simulink model "pwm_fpga"  (R2020b)
settings: Solver=FixedStepDiscrete  StartTime=0.0  StopTime=5  FixedStep=1e-3  RelTol=1e-3
PostLoadFcn:
  | try
  | cell = struct2cell(dir(fullfile(speedgoatroot_hdlb, 'hdlsrc', 'pwm', '*.vhd')));
  | addSourceFiles = strjoin(fullfile(cell(2,:),cell(1,:)), ';');
  | hdlset_param('pwm_example_hdlc/DUT PWM and CAP', 'IPCoreAdditionalFiles', addSourceFiles);
  | end
libraries: pwm_fpgalib x1, pwm_cpulib x1
settings Model: ModifiedByFormat=Speedgoat GmbH  Creator=Speedgoat GmbH  LastModifiedBy=Speedgoat GmbH
settings DataIOCC: LimitDataPoints=on  SaveFormat=Array  ReturnWorkspaceOutputs=off
settings OptimizationCC: BlockReduction=off  ConditionallyExecuteInputs=off  DefaultParameterBehavior=Inlined  LifeSpan=inf
settings DebuggingCC: AlgebraicLoopMsg=error  UnderspecifiedInitializationDetection=Classic  MergeDetectMultiDrivingBlocksExec=none  SolverPrmCheckMsg=warning  SingleTaskRateTransMsg=error  PregeneratedLibrarySubsystemCodeDiagnostic=none  SFUnexpectedBacktrackingDiag=warning  SFNoUnconditionalDefaultTransitionDiag=warning  SFExecutionAtInitializationDiag=none  ArithmeticOperatorsInVariantConditions=warning
settings HardwareCC: ProdBitPerPointer=32  ProdBitPerSizeT=32  ProdBitPerPtrDiffT=32  ProdLargestAtomicFloat=None  ProdIntDivRoundTo=Undefined  ProdEndianess=Unspecified  ProdWordSize=32  ProdHWDeviceType=ASIC/FPGA->ASIC/FPGA  ProdEqTarget=off
settings ModelReferenceCC: PropagateSignalLabelsOutOfModel=off
settings SFSimCC: SimUseLocalCustomCode=off  CustomCodeUndefinedFunction=UseInterfaceOnly
settings RTWCC: RTWUseLocalCustomCode=off
settings CodeAppCC: StateflowObjectComments=on
settings GRTTargetCC: TargetLangStandard=C89/C90 (ANSI)
settings ConfigComp: CovMetricSettings=dw  CovSaveCumulativeToWorkspaceVar=on  CovSaveSingleToWorkspaceVar=on  CovExternalEMLEnable=off

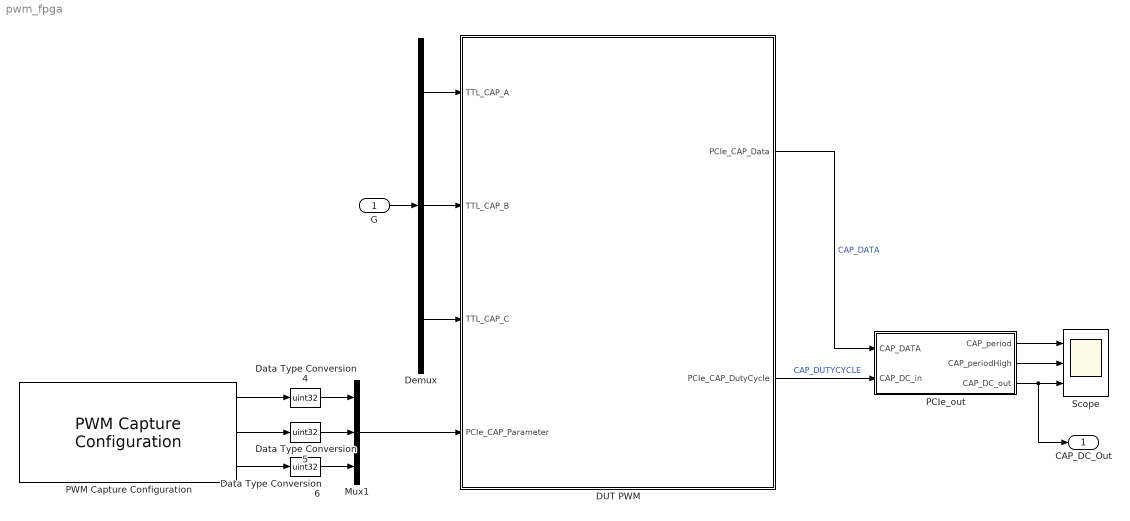
== system pwm_fpga ==
  G : Inport
  DUT PWM : Subsystem
  Data Type Conversion4 : DataTypeConversion  OutDataTypeStr=uint32
  Data Type Conversion5 : DataTypeConversion  OutDataTypeStr=uint32
  Data Type Conversion6 : DataTypeConversion  OutDataTypeStr=uint32
  Demux : Demux  Outputs=3
  Mux1 : Mux  Inputs=3
  PCIe_out : Subsystem
  PWM Capture Configuration : pwm_cpulib/PWM Capture Configuration  FPGA_freq=100e6  n_channels=1  captureMode=High transitions triggered  captureTimeout=0  PWM_pattern_en=off
      settings: SourceProductName=Simulink Real-Time: Speedgoat HDL Blockset
  Scope : Scope  NumInputPorts=3
  CAP_DC_Out : Outport  VectorParamsAs1DForOutWhenUnconnected=off
  wires:
  DUT PWM/2(PCIe_CAP_DutyCycle) -> PCIe_out/2(CAP_DC_in)  "CAP_DUTYCYCLE"
  DUT PWM/1(PCIe_CAP_Data) -> PCIe_out/1(CAP_DATA)  "CAP_DATA"
  PCIe_out/3(CAP_DC_out) -> Scope/3, CAP_DC_Out/1
  PCIe_out/2(CAP_periodHigh) -> Scope/2
  PCIe_out/1(CAP_period) -> Scope/1
  PWM Capture Configuration/1 -> Data Type Conversion4/1
  PWM Capture Configuration/3 -> Data Type Conversion6/1
  PWM Capture Configuration/2 -> Data Type Conversion5/1
  Data Type Conversion4/1 -> Mux1/1
  Data Type Conversion5/1 -> Mux1/2
  Data Type Conversion6/1 -> Mux1/3
  Mux1/1 -> DUT PWM/4(PCIe_CAP_Parameter)
  Demux/1 -> DUT PWM/1(TTL_CAP_A)
  Demux/3 -> DUT PWM/3(TTL_CAP_C)
  Demux/2 -> DUT PWM/2(TTL_CAP_B)
  G/1 -> Demux/1

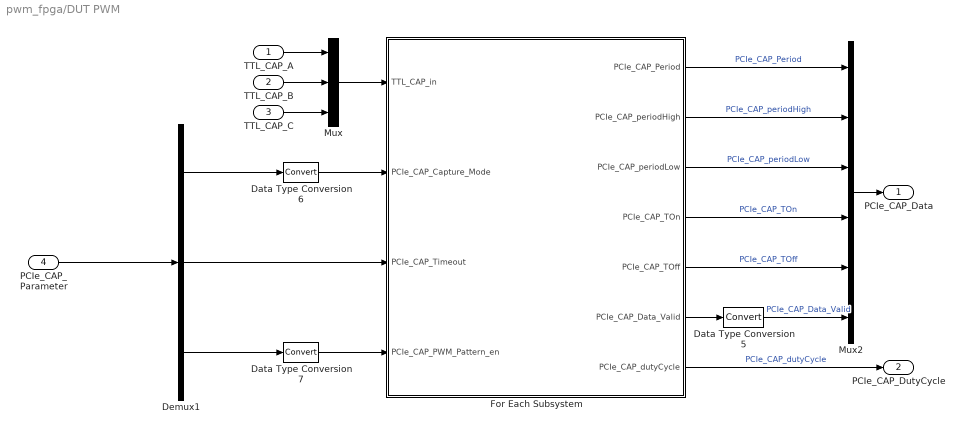
== system pwm_fpga/DUT PWM ==
  TTL_CAP_A : Inport
  TTL_CAP_B : Inport  Port=2
  TTL_CAP_C : Inport  Port=3
  PCIe_CAP_Parameter : Inport  Port=4
  Data Type Conversion5 : DataTypeConversion
  Data Type Conversion6 : DataTypeConversion
  Data Type Conversion7 : DataTypeConversion
  Demux1 : Demux  Outputs=3
  For Each Subsystem : Subsystem  TreatAsAtomicUnit=on
  Mux : Mux  Inputs=3
  Mux2 : Mux  Inputs=6
  PCIe_CAP_Data : Outport  VectorParamsAs1DForOutWhenUnconnected=off
  PCIe_CAP_DutyCycle : Outport  Port=2  VectorParamsAs1DForOutWhenUnconnected=off
  wires:
  Demux1/1 -> Data Type Conversion6/1
  TTL_CAP_A/1 -> Mux/1
  For Each Subsystem/7(PCIe_CAP_dutyCycle) -> PCIe_CAP_DutyCycle/1  "PCIe_CAP_dutyCycle"
  Demux1/2 -> For Each Subsystem/3(PCIe_CAP_Timeout)
  Demux1/3 -> Data Type Conversion7/1
  For Each Subsystem/6(PCIe_CAP_Data_Valid) -> Data Type Conversion5/1
  For Each Subsystem/5(PCIe_CAP_TOff) -> Mux2/5  "PCIe_CAP_TOff"
  For Each Subsystem/4(PCIe_CAP_TOn) -> Mux2/4  "PCIe_CAP_TOn"
  For Each Subsystem/3(PCIe_CAP_periodLow) -> Mux2/3  "PCIe_CAP_periodLow"
  For Each Subsystem/1(PCIe_CAP_Period) -> Mux2/1  "PCIe_CAP_Period"
  For Each Subsystem/2(PCIe_CAP_periodHigh) -> Mux2/2  "PCIe_CAP_periodHigh"
  Mux/1 -> For Each Subsystem/1(TTL_CAP_in)
  TTL_CAP_B/1 -> Mux/2
  Mux2/1 -> PCIe_CAP_Data/1
  Data Type Conversion5/1 -> Mux2/6  "PCIe_CAP_Data_Valid"
  PCIe_CAP_Parameter/1 -> Demux1/1
  Data Type Conversion6/1 -> For Each Subsystem/2(PCIe_CAP_Capture_Mode)
  Data Type Conversion7/1 -> For Each Subsystem/4(PCIe_CAP_PWM_Pattern_en)
  TTL_CAP_C/1 -> Mux/3

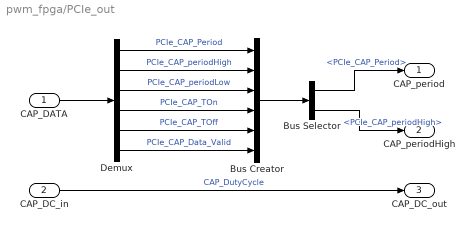
== system pwm_fpga/PCIe_out ==
  CAP_DATA : Inport
  CAP_DC_in : Inport  Port=2
  Bus Creator : BusCreator  Inputs=6
  Bus Selector : BusSelector  OutputSignals=PCIe_CAP_Period,PCIe_CAP_periodHigh
  Demux : Demux  Outputs=6
  CAP_period : Outport
  CAP_periodHigh : Outport  Port=2
  CAP_DC_out : Outport  Port=3
  wires:
  CAP_DC_in/1 -> CAP_DC_out/1  "CAP_DutyCycle"
  Bus Selector/2 -> CAP_periodHigh/1  "<PCIe_CAP_periodHigh>"
  Bus Selector/1 -> CAP_period/1  "<PCIe_CAP_Period>"
  Demux/6 -> Bus Creator/6  "PCIe_CAP_Data_Valid"
  Demux/3 -> Bus Creator/3  "PCIe_CAP_periodLow"
  Demux/2 -> Bus Creator/2  "PCIe_CAP_periodHigh"
  Demux/4 -> Bus Creator/4  "PCIe_CAP_TOn"
  Bus Creator/1 -> Bus Selector/1
  Demux/1 -> Bus Creator/1  "PCIe_CAP_Period"
  Demux/5 -> Bus Creator/5  "PCIe_CAP_TOff"
  CAP_DATA/1 -> Demux/1

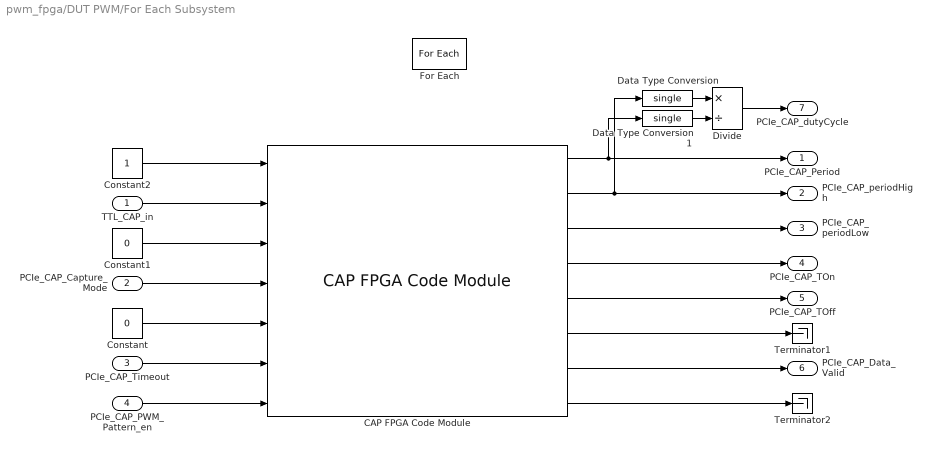
== system pwm_fpga/DUT PWM/For Each Subsystem ==
  TTL_CAP_in : Inport  Partition=on  PartitionDimension=1  PartitionWidth=1  PartitionOffset=0
  PCIe_CAP_Capture_Mode : Inport  Port=2
  PCIe_CAP_Timeout : Inport  Port=3
  PCIe_CAP_PWM_Pattern_en : Inport  Port=4
  CAP FPGA Code Module : pwm_fpgalib/CAP FPGA Code Module  SystemSampleTime=-1  VariantActivationTime=update diagram  Latency=0  AutoFrameSizeCalculation=off
      settings: SourceProductName=Simulink Real-Time: Speedgoat Functionality Package
  Constant : Constant  Value=0  OutDataTypeStr=Inherit: Inherit via back propagation  SampleTime=-1
  Constant1 : Constant  Value=0  OutDataTypeStr=Inherit: Inherit via back propagation  SampleTime=-1
  Constant2 : Constant  OutDataTypeStr=Inherit: Inherit via back propagation  SampleTime=-1
  Data Type Conversion : DataTypeConversion  OutMin=0  OutDataTypeStr=single
  Data Type Conversion1 : DataTypeConversion  OutMin=0  OutDataTypeStr=single  LockScale=on
  Divide : Product  Inputs=*/  RndMeth=Zero  SaturateOnIntegerOverflow=on
  For Each : ForEach  DisableCoverage=on
  Terminator1 : Terminator
  Terminator2 : Terminator
  PCIe_CAP_Period : Outport  ConcatenationDimension=2  VectorParamsAs1DForOutWhenUnconnected=off
  PCIe_CAP_periodHigh : Outport  Port=2  ConcatenationDimension=2  VectorParamsAs1DForOutWhenUnconnected=off
  PCIe_CAP_periodLow : Outport  Port=3  ConcatenationDimension=2  VectorParamsAs1DForOutWhenUnconnected=off
  PCIe_CAP_TOn : Outport  Port=4  ConcatenationDimension=2  VectorParamsAs1DForOutWhenUnconnected=off
  PCIe_CAP_TOff : Outport  Port=5  ConcatenationDimension=2  VectorParamsAs1DForOutWhenUnconnected=off
  PCIe_CAP_Data_Valid : Outport  Port=6  ConcatenationDimension=2  VectorParamsAs1DForOutWhenUnconnected=off
  PCIe_CAP_dutyCycle : Outport  Port=7  ConcatenationDimension=2  VectorParamsAs1DForOutWhenUnconnected=off
  wires:
  Data Type Conversion/1 -> Divide/1
  Divide/1 -> PCIe_CAP_dutyCycle/1
  Constant1/1 -> CAP FPGA Code Module/3
  PCIe_CAP_Capture_Mode/1 -> CAP FPGA Code Module/4
  Constant/1 -> CAP FPGA Code Module/5
  TTL_CAP_in/1 -> CAP FPGA Code Module/2
  PCIe_CAP_Timeout/1 -> CAP FPGA Code Module/6
  PCIe_CAP_PWM_Pattern_en/1 -> CAP FPGA Code Module/7
  Constant2/1 -> CAP FPGA Code Module/1
  CAP FPGA Code Module/3 -> PCIe_CAP_periodLow/1
  CAP FPGA Code Module/8 -> Terminator2/1
  CAP FPGA Code Module/5 -> PCIe_CAP_TOff/1
  CAP FPGA Code Module/6 -> Terminator1/1
  CAP FPGA Code Module/2 -> PCIe_CAP_periodHigh/1, Data Type Conversion/1
  CAP FPGA Code Module/7 -> PCIe_CAP_Data_Valid/1
  CAP FPGA Code Module/1 -> PCIe_CAP_Period/1, Data Type Conversion1/1
  CAP FPGA Code Module/4 -> PCIe_CAP_TOn/1
  Data Type Conversion1/1 -> Divide/2
